simulink model "Basic_DMT"  (R2014b)
settings: Solver=FixedStepDiscrete  SolverMode=SingleTasking  StartTime=0.0  StopTime=25e-6-14e-9*24  RelTol=1e-3
PreLoadFcn:
  | userName = getenv('UserName');
  | 
  | if strcmp(userName,'Tim')
  | cd C:\Users\Tim\Documents\GitHub\MA_1\Basic_DMT
  | else
  | cd C:\Users\Tim-UML\Documents\GitHub\MA_1\Basic_DMT
  | end
InitFcn:
  | userName = getenv('UserName');
  | 
  | if strcmp(userName,'Tim')
  | cd C:\Users\Tim\Documents\GitHub\MA_1\Basic_DMT
  | else
  | cd C:\Users\Tim-UML\Documents\GitHub\MA_1\Basic_DMT
  | end
values from neighbouring files (symbols this model uses):
  a0 = 0.21194908595403703    (= 0.211949085954)    [initScript.m]
  a1 = 0.576101828091926    (= 0.576101828092)    [initScript.m]
  a2 = a0    (= 0.211949085954)    [initScript.m]
  beta = 1    [initScript.m]
  bitPerSymb = 4    [initScript.m]
  chanDownFact = Tchan/SystemPeriod    [initScript.m]
  fftLen = 16    [initScript.m]
  fftLenActive = fftLenDMT    (= 32)    [initScript.m]
  fftLenDMT = 2*fftLen    (= 32)    [initScript.m]
  GI_Active = GI_LenDMT    (= 0)    [initScript.m]
  GI_Len = 0    [initScript.m]
  GI_LenDMT = 0    [initScript.m]
  M = log2(fftLen)    [initScript.m]
  sysgenSystemPeriod = 4e-9    (= 4e-09)    [initScript.m]
  SystemPeriod = 4e-9    (= 4e-09)    [initScript.m]
  upsampleFactor = 1    [initScript.m]
  usedSubCar = 14    [initScript.m]
undefined symbols (not defined in the file or in its folder): bitCount, get, modu_mode, Tb, Ts
libraries: xbsIndex_r4 x822, commdigbbndam3 x59, simulink x42, dspsigops x7, commrandsrc2 x6, dspbuff3 x4, dspxfrm3 x3, dspswit3 x2, commseqgen2 x1, dsparch4 x1, commutil2 x1, dspsnks4 x1
(part 3 of 10)

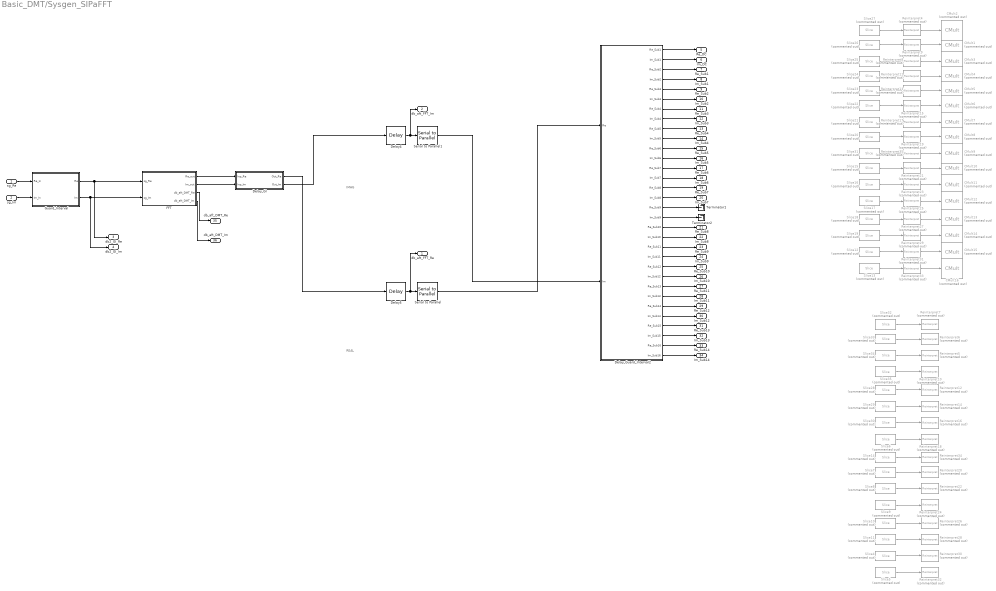
== system Basic_DMT/Sysgen_SIPaFFT ==
  note: IMAG
  note: REAL
  sg_Re : Inport
  sg_Im : Inport  Port=2
  CMult1 : xbsIndex_r4/CMult  Commented=on  const=1/e10  gui_display_data_type=Fixed-point  const_n_bits=bitCount+(log2(fftLen)+1)*2  const_bin_pt=fracLen  float_type=Single  exp_bits=8  fraction_bits=24  en=off  latency=0  precision=User Defined  arith_type="Signed  (2's comp)"  n_bits=bitCount+(log2(fftLen)+1)*2  bin_pt=fracLen  quantization="Round  (unbiased: +/- Inf)"  overflow=Saturate  use_behavioral_HDL=off  mem_type=Distributed RAM  pipeline=off  dbl_ovrd=off  block_type=cmult
  CMult{2,6..16} (12 alike) : xbsIndex_r4/CMult  Commented=on  const=1/e9  gui_display_data_type=Fixed-point  const_n_bits=bitCount+(log2(fftLen)+1)*2  const_bin_pt=fracLen  float_type=Single  exp_bits=8  fraction_bits=24  en=off  latency=0  precision=User Defined  arith_type="Signed  (2's comp)"  n_bits=bitCount+(log2(fftLen)+1)*2  bin_pt=fracLen  quantization="Round  (unbiased: +/- Inf)"  overflow=Saturate  use_behavioral_HDL=off  mem_type=Distributed RAM  pipeline=off  dbl_ovrd=off  block_type=cmult
  CMult3 : xbsIndex_r4/CMult  Commented=on  const=1/e11  gui_display_data_type=Fixed-point  const_n_bits=bitCount+(log2(fftLen)+1)*2  const_bin_pt=fracLen  float_type=Single  exp_bits=8  fraction_bits=24  en=off  latency=0  precision=User Defined  arith_type="Signed  (2's comp)"  n_bits=bitCount+(log2(fftLen)+1)*2  bin_pt=fracLen  quantization="Round  (unbiased: +/- Inf)"  overflow=Saturate  use_behavioral_HDL=off  mem_type=Distributed RAM  pipeline=off  dbl_ovrd=off  block_type=cmult
  CMult4 : xbsIndex_r4/CMult  Commented=on  const=1/e12  gui_display_data_type=Fixed-point  const_n_bits=bitCount+(log2(fftLen)+1)*2  const_bin_pt=fracLen  float_type=Single  exp_bits=8  fraction_bits=24  en=off  latency=0  precision=User Defined  arith_type="Signed  (2's comp)"  n_bits=bitCount+(log2(fftLen)+1)*2  bin_pt=fracLen  quantization="Round  (unbiased: +/- Inf)"  overflow=Saturate  use_behavioral_HDL=off  mem_type=Distributed RAM  pipeline=off  dbl_ovrd=off  block_type=cmult
  CMult5 : xbsIndex_r4/CMult  Commented=on  const=1/e13  gui_display_data_type=Fixed-point  const_n_bits=bitCount+(log2(fftLen)+1)*2  const_bin_pt=fracLen  float_type=Single  exp_bits=8  fraction_bits=24  en=off  latency=0  precision=User Defined  arith_type="Signed  (2's comp)"  n_bits=bitCount+(log2(fftLen)+1)*2  bin_pt=fracLen  quantization="Round  (unbiased: +/- Inf)"  overflow=Saturate  use_behavioral_HDL=off  mem_type=Distributed RAM  pipeline=off  dbl_ovrd=off  block_type=cmult
  Delay4 : xbsIndex_r4/Delay  rst=off  infoeditControl=Selection of Reset will increase slice count due to use of real FFs and instead of SRLs  en=off  latency=4  reg_retiming=off  dbl_ovrd=off  block_type=delay
  Delay5 : xbsIndex_r4/Delay  rst=off  infoeditControl=Selection of Reset will increase slice count due to use of real FFs and instead of SRLs  en=off  latency=4  reg_retiming=off  dbl_ovrd=off  block_type=delay
  Delay_GI : Subsystem  Variant=on
  Delay_Guard_Interval2 : Subsystem  Variant=on
  FFT : Subsystem  Variant=on
  Guard_Interval : Subsystem  Variant=on
  Reinterpret{4..35} (32 alike) : xbsIndex_r4/Reinterpret  Commented=on  force_arith_type=on  arith_type="Signed  (2's comp)"  force_bin_pt=on  bin_pt=fracLen  block_type=reinterpret
  Serial to Parallel : xbsIndex_r4/Serial to Parallel  input_order=Most Significant Word First  arith_type=Unsigned  output_bits=(bitCount+(log2(fftLen)+1)*2)*fftLen  bin_pt=0  rst=off  en=off  latency=1  dbl_ovrd=off  block_type=s2p
      settings: infoedit=Groups of samples presented serially at the input become single samples presented at the output.
  Serial to Parallel1 : xbsIndex_r4/Serial to Parallel  input_order=Most Significant Word First  arith_type=Unsigned  output_bits=(bitCount+(log2(fftLen)+1)*2)*fftLen  bin_pt=0  rst=off  en=off  latency=1  dbl_ovrd=off  block_type=s2p
      settings: infoedit=Groups of samples presented serially at the input become single samples presented at the output.
  Slice10 : xbsIndex_r4/Slice  Commented=on  nbits=(bitCount+(log2(fftLen)+1)*2)  boolean_output=off  mode=Lower Bit Location + Width  bit1=0  base1=MSB of Input  bit0=(bitCount+(log2(fftLen)+1)*2)*3  base0=LSB of Input  dbl_ovrd=off  block_type=slice
  Slice11 : xbsIndex_r4/Slice  Commented=on  nbits=(bitCount+(log2(fftLen)+1)*2)  boolean_output=off  mode=Lower Bit Location + Width  bit1=0  base1=MSB of Input  bit0=(bitCount+(log2(fftLen)+1)*2)*2  base0=LSB of Input  dbl_ovrd=off  block_type=slice
  Slice12 : xbsIndex_r4/Slice  Commented=on  nbits=(bitCount+(log2(fftLen)+1)*2)  boolean_output=off  mode=Lower Bit Location + Width  bit1=0  base1=MSB of Input  bit0=(bitCount+(log2(fftLen)+1)*2)*1  base0=LSB of Input  dbl_ovrd=off  block_type=slice
  Slice13 : xbsIndex_r4/Slice  Commented=on  nbits=(bitCount+(log2(fftLen)+1)*2)  boolean_output=off  mode=Lower Bit Location + Width  bit1=0  base1=MSB of Input  bit0=0  base0=LSB of Input  dbl_ovrd=off  block_type=slice
  Slice14 : xbsIndex_r4/Slice  Commented=on  nbits=(bitCount+(log2(fftLen)+1)*2)  boolean_output=off  mode=Lower Bit Location + Width  bit1=0  base1=LSB of Input  bit0=(bitCount+(log2(fftLen)+1)*2)*7  base0=LSB of Input  dbl_ovrd=off  block_type=slice
  Slice15 : xbsIndex_r4/Slice  Commented=on  nbits=(bitCount+(log2(fftLen)+1)*2)  boolean_output=off  mode=Lower Bit Location + Width  bit1=24  base1=LSB of Input  bit0=(bitCount+(log2(fftLen)+1)*2)*6  base0=LSB of Input  dbl_ovrd=off  block_type=slice
  Slice16 : xbsIndex_r4/Slice  Commented=on  nbits=(bitCount+(log2(fftLen)+1)*2)  boolean_output=off  mode=Lower Bit Location + Width  bit1=0  base1=MSB of Input  bit0=(bitCount+(log2(fftLen)+1)*2)*5  base0=LSB of Input  dbl_ovrd=off  block_type=slice
  Slice17 : xbsIndex_r4/Slice  Commented=on  nbits=(bitCount+(log2(fftLen)+1)*2)  boolean_output=off  mode=Lower Bit Location + Width  bit1=0  base1=MSB of Input  bit0=(bitCount+(log2(fftLen)+1)*2)*4  base0=LSB of Input  dbl_ovrd=off  block_type=slice
  Slice18 : xbsIndex_r4/Slice  Commented=on  nbits=(bitCount+(log2(fftLen)+1)*2)  boolean_output=off  mode=Lower Bit Location + Width  bit1=0  base1=MSB of Input  bit0=(bitCount+(log2(fftLen)+1)*2)*3  base0=LSB of Input  dbl_ovrd=off  block_type=slice
  Slice19 : xbsIndex_r4/Slice  Commented=on  nbits=(bitCount+(log2(fftLen)+1)*2)  boolean_output=off  mode=Lower Bit Location + Width  bit1=0  base1=MSB of Input  bit0=(bitCount+(log2(fftLen)+1)*2)*2  base0=LSB of Input  dbl_ovrd=off  block_type=slice
  Slice20 : xbsIndex_r4/Slice  Commented=on  nbits=(bitCount+(log2(fftLen)+1)*2)  boolean_output=off  mode=Lower Bit Location + Width  bit1=0  base1=LSB of Input  bit0=(bitCount+(log2(fftLen)+1)*2)*8  base0=LSB of Input  dbl_ovrd=off  block_type=slice
  Slice21 : xbsIndex_r4/Slice  Commented=on  nbits=(bitCount+(log2(fftLen)+1)*2)  boolean_output=off  mode=Lower Bit Location + Width  bit1=0  base1=LSB of Input  bit0=(bitCount+(log2(fftLen)+1)*2)*9  base0=LSB of Input  dbl_ovrd=off  block_type=slice
  Slice22 : xbsIndex_r4/Slice  Commented=on  nbits=(bitCount+(log2(fftLen)+1)*2)  boolean_output=off  mode=Lower Bit Location + Width  bit1=0  base1=LSB of Input  bit0=(bitCount+(log2(fftLen)+1)*2)*10  base0=LSB of Input  dbl_ovrd=off  block_type=slice
  Slice23 : xbsIndex_r4/Slice  Commented=on  nbits=(bitCount+(log2(fftLen)+1)*2)  boolean_output=off  mode=Lower Bit Location + Width  bit1=0  base1=LSB of Input  bit0=(bitCount+(log2(fftLen)+1)*2)*11  base0=LSB of Input  dbl_ovrd=off  block_type=slice
  Slice24 : xbsIndex_r4/Slice  Commented=on  nbits=(bitCount+(log2(fftLen)+1)*2)  boolean_output=off  mode=Lower Bit Location + Width  bit1=0  base1=LSB of Input  bit0=(bitCount+(log2(fftLen)+1)*2)*12  base0=LSB of Input  dbl_ovrd=off  block_type=slice
  Slice25 : xbsIndex_r4/Slice  Commented=on  nbits=(bitCount+(log2(fftLen)+1)*2)  boolean_output=off  mode=Lower Bit Location + Width  bit1=0  base1=LSB of Input  bit0=(bitCount+(log2(fftLen)+1)*2)*13  base0=LSB of Input  dbl_ovrd=off  block_type=slice
  Slice26 : xbsIndex_r4/Slice  Commented=on  nbits=(bitCount+(log2(fftLen)+1)*2)  boolean_output=off  mode=Lower Bit Location + Width  bit1=0  base1=LSB of Input  bit0=(bitCount+(log2(fftLen)+1)*2)*14  base0=LSB of Input  dbl_ovrd=off  block_type=slice
  Slice27 : xbsIndex_r4/Slice  Commented=on  nbits=(bitCount+(log2(fftLen)+1)*2)  boolean_output=off  mode=Lower Bit Location + Width  bit1=0  base1=LSB of Input  bit0=(bitCount+(log2(fftLen)+1)*2)*15  base0=LSB of Input  dbl_ovrd=off  block_type=slice
  Slice28 : xbsIndex_r4/Slice  Commented=on  nbits=(bitCount+(log2(fftLen)+1)*2)  boolean_output=off  mode=Lower Bit Location + Width  bit1=0  base1=MSB of Input  bit0=(bitCount+(log2(fftLen)+1)*2)*11  base0=LSB of Input  dbl_ovrd=off  block_type=slice
  Slice29 : xbsIndex_r4/Slice  Commented=on  nbits=(bitCount+(log2(fftLen)+1)*2)  boolean_output=off  mode=Lower Bit Location + Width  bit1=0  base1=MSB of Input  bit0=(bitCount+(log2(fftLen)+1)*2)*10  base0=LSB of Input  dbl_ovrd=off  block_type=slice
  Slice30 : xbsIndex_r4/Slice  Commented=on  nbits=(bitCount+(log2(fftLen)+1)*2)  boolean_output=off  mode=Lower Bit Location + Width  bit1=0  base1=MSB of Input  bit0=(bitCount+(log2(fftLen)+1)*2)*9  base0=LSB of Input  dbl_ovrd=off  block_type=slice
  Slice31 : xbsIndex_r4/Slice  Commented=on  nbits=(bitCount+(log2(fftLen)+1)*2)  boolean_output=off  mode=Lower Bit Location + Width  bit1=0  base1=LSB of Input  bit0=(bitCount+(log2(fftLen)+1)*2)*7  base0=LSB of Input  dbl_ovrd=off  block_type=slice
  Slice32 : xbsIndex_r4/Slice  Commented=on  nbits=(bitCount+(log2(fftLen)+1)*2)  boolean_output=off  mode=Lower Bit Location + Width  bit1=0  base1=LSB of Input  bit0=(bitCount+(log2(fftLen)+1)*2)*15  base0=LSB of Input  dbl_ovrd=off  block_type=slice
  Slice33 : xbsIndex_r4/Slice  Commented=on  nbits=(bitCount+(log2(fftLen)+1)*2)  boolean_output=off  mode=Lower Bit Location + Width  bit1=24  base1=LSB of Input  bit0=(bitCount+(log2(fftLen)+1)*2)*14  base0=LSB of Input  dbl_ovrd=off  block_type=slice
  Slice34 : xbsIndex_r4/Slice  Commented=on  nbits=(bitCount+(log2(fftLen)+1)*2)  boolean_output=off  mode=Lower Bit Location + Width  bit1=0  base1=MSB of Input  bit0=(bitCount+(log2(fftLen)+1)*2)*13  base0=LSB of Input  dbl_ovrd=off  block_type=slice
  Slice35 : xbsIndex_r4/Slice  Commented=on  nbits=(bitCount+(log2(fftLen)+1)*2)  boolean_output=off  mode=Lower Bit Location + Width  bit1=0  base1=MSB of Input  bit0=(bitCount+(log2(fftLen)+1)*2)*12  base0=LSB of Input  dbl_ovrd=off  block_type=slice
  Slice4 : xbsIndex_r4/Slice  Commented=on  nbits=(bitCount+(log2(fftLen)+1)*2)  boolean_output=off  mode=Lower Bit Location + Width  bit1=0  base1=MSB of Input  bit0=(bitCount+(log2(fftLen)+1)*2)  base0=LSB of Input  dbl_ovrd=off  block_type=slice
  Slice5 : xbsIndex_r4/Slice  Commented=on  nbits=(bitCount+(log2(fftLen)+1)*2)  boolean_output=off  mode=Lower Bit Location + Width  bit1=0  base1=MSB of Input  bit0=0  base0=LSB of Input  dbl_ovrd=off  block_type=slice
  Slice6 : xbsIndex_r4/Slice  Commented=on  nbits=(bitCount+(log2(fftLen)+1)*2)  boolean_output=off  mode=Lower Bit Location + Width  bit1=0  base1=LSB of Input  bit0=(bitCount+(log2(fftLen)+1)*2)*8  base0=LSB of Input  dbl_ovrd=off  block_type=slice
  Slice7 : xbsIndex_r4/Slice  Commented=on  nbits=(bitCount+(log2(fftLen)+1)*2)  boolean_output=off  mode=Lower Bit Location + Width  bit1=24  base1=LSB of Input  bit0=(bitCount+(log2(fftLen)+1)*2)*6  base0=LSB of Input  dbl_ovrd=off  block_type=slice
  Slice8 : xbsIndex_r4/Slice  Commented=on  nbits=(bitCount+(log2(fftLen)+1)*2)  boolean_output=off  mode=Lower Bit Location + Width  bit1=0  base1=MSB of Input  bit0=(bitCount+(log2(fftLen)+1)*2)*5  base0=LSB of Input  dbl_ovrd=off  block_type=slice
  Slice9 : xbsIndex_r4/Slice  Commented=on  nbits=(bitCount+(log2(fftLen)+1)*2)  boolean_output=off  mode=Lower Bit Location + Width  bit1=0  base1=MSB of Input  bit0=(bitCount+(log2(fftLen)+1)*2)*4  base0=LSB of Input  dbl_ovrd=off  block_type=slice
  Terminator1 : Terminator
  Terminator2 : Terminator
  db_aft_FFT_Re : Outport
  db_aft_FFT_Im : Outport  Port=2
  db2_GI_Re : Outport  Port=3
  db2_GI_Im : Outport  Port=4
  Re_DC : Outport  Port=5
  Im_DC : Outport  Port=6
  Re_Sub1 : Outport  Port=7
  Im_Sub1 : Outport  Port=8
  Re_Sub2 : Outport  Port=9
  Im_Sub2 : Outport  Port=10
  Re_Sub3 : Outport  Port=11
  Im_Sub3 : Outport  Port=12
  Re_Sub4 : Outport  Port=13
  Im_Sub4 : Outport  Port=14
  Re_Sub5 : Outport  Port=15
  Im_Sub5 : Outport  Port=16
  Re_Sub6 : Outport  Port=17
  Im_Sub6 : Outport  Port=18
  Re_Sub7 : Outport  Port=19
  Im_Sub7 : Outport  Port=20
  Re_Sub8 : Outport  Port=21
  Im_Sub8 : Outport  Port=22
  Re_Sub9 : Outport  Port=23
  Im_Sub9 : Outport  Port=24
  Re_Sub10 : Outport  Port=25
  Im_Sub10 : Outport  Port=26
  Re_Sub11 : Outport  Port=27
  Im_Sub11 : Outport  Port=28
  Re_Sub12 : Outport  Port=29
  Im_Sub12 : Outport  Port=30
  Re_Sub13 : Outport  Port=31
  Im_Sub13 : Outport  Port=32
  Re_Sub14 : Outport  Port=33
  Im_Sub14 : Outport  Port=34
  db_aft_DMT_Re : Outport  Port=35
  db_aft_DMT_Im : Outport  Port=36
  wires:
  Delay_Guard_Interval2/1(Re_Sub1) -> Re_DC/1
  Delay_Guard_Interval2/3(Re_Sub2) -> Re_Sub1/1
  Delay4/1 -> db_aft_FFT_Im/1, Serial to Parallel1/1
  Delay5/1 -> db_aft_FFT_Re/1, Serial to Parallel/1
  Delay_Guard_Interval2/5(Re_Sub3) -> Re_Sub2/1
  Guard_Interval/1(Re) -> FFT/1(sg_Re), db2_GI_Re/1
  Guard_Interval/2(Im) -> FFT/2(sg_Im), db2_GI_Im/1
  sg_Im/1 -> Guard_Interval/2(Im_In)
  sg_Re/1 -> Guard_Interval/1(Re_In)
  Delay_Guard_Interval2/7(Re_Sub4) -> Re_Sub3/1
  Delay_Guard_Interval2/9(Re_Sub5) -> Re_Sub4/1
  Delay_Guard_Interval2/11(Re_Sub6) -> Re_Sub5/1
  Delay_Guard_Interval2/15(Re_Sub8) -> Re_Sub7/1
  Delay_Guard_Interval2/13(Re_Sub7) -> Re_Sub6/1
  Delay_Guard_Interval2/23(Re_Sub12) -> Re_Sub10/1
  Delay_Guard_Interval2/19(Re_Sub10) -> Re_Sub8/1
  Delay_Guard_Interval2/21(Re_Sub11) -> Re_Sub9/1
  Delay_Guard_Interval2/25(Re_Sub13) -> Re_Sub11/1
  Delay_Guard_Interval2/27(Re_Sub14) -> Re_Sub12/1
  Delay_Guard_Interval2/29(Re_Sub15) -> Re_Sub13/1
  Delay_Guard_Interval2/31(Re_Sub16) -> Re_Sub14/1
  Serial to Parallel/1 -> Delay_Guard_Interval2/1(Re)
  Delay_Guard_Interval2/17(Re_Sub9) -> Terminator1/1
  Delay_GI/2(Out_Im) -> Delay4/1
  Delay_GI/1(Out_Re) -> Delay5/1
  FFT/3(db_aft_DMT_Re) -> db_aft_DMT_Re/1
  FFT/4(db_aft_DMT_Im) -> db_aft_DMT_Im/1
  FFT/1(Re_out) -> Delay_GI/1(Inp_Re)
  FFT/2(Im_out) -> Delay_GI/2(Inp_Im)
  Delay_Guard_Interval2/2(Im_Sub1) -> Im_DC/1
  Delay_Guard_Interval2/4(Im_Sub2) -> Im_Sub1/1
  Delay_Guard_Interval2/6(Im_Sub3) -> Im_Sub2/1
  Delay_Guard_Interval2/8(Im_Sub4) -> Im_Sub3/1
  Delay_Guard_Interval2/10(Im_Sub5) -> Im_Sub4/1
  Delay_Guard_Interval2/12(Im_Sub6) -> Im_Sub5/1
  Delay_Guard_Interval2/14(Im_Sub7) -> Im_Sub6/1
  Delay_Guard_Interval2/16(Im_Sub8) -> Im_Sub7/1
  Delay_Guard_Interval2/18(Im_Sub9) -> Terminator2/1
  Delay_Guard_Interval2/20(Im_Sub10) -> Im_Sub8/1
  Delay_Guard_Interval2/22(Im_Sub11) -> Im_Sub9/1
  Delay_Guard_Interval2/24(Im_Sub12) -> Im_Sub10/1
  Delay_Guard_Interval2/26(Im_Sub13) -> Im_Sub11/1
  Delay_Guard_Interval2/28(Im_Sub14) -> Im_Sub12/1
  Delay_Guard_Interval2/30(Im_Sub15) -> Im_Sub13/1
  Delay_Guard_Interval2/32(Im_Sub16) -> Im_Sub14/1
  Reinterpret4/1 -> CMult2/1
  Reinterpret9/1 -> CMult1/1
  Reinterpret8/1 -> CMult3/1
  Slice26/1 -> Reinterpret9/1
  Slice27/1 -> Reinterpret4/1
  Reinterpret11/1 -> CMult4/1
  Reinterpret13/1 -> CMult5/1
  Reinterpret15/1 -> CMult6/1
  Reinterpret17/1 -> CMult7/1
  Reinterpret19/1 -> CMult8/1
  Reinterpret21/1 -> CMult10/1
  Reinterpret23/1 -> CMult11/1
  Reinterpret25/1 -> CMult12/1
  Reinterpret27/1 -> CMult13/1
  Reinterpret29/1 -> CMult14/1
  Reinterpret31/1 -> CMult15/1
  Reinterpret33/1 -> CMult16/1
  Slice25/1 -> Reinterpret8/1
  Slice24/1 -> Reinterpret11/1
  Slice23/1 -> Reinterpret13/1
  Slice22/1 -> Reinterpret15/1
  Slice20/1 -> Reinterpret19/1
  Slice21/1 -> Reinterpret17/1
  Slice15/1 -> Reinterpret21/1
  Slice16/1 -> Reinterpret23/1
  Slice17/1 -> Reinterpret25/1
  Slice18/1 -> Reinterpret27/1
  Slice19/1 -> Reinterpret29/1
  Slice12/1 -> Reinterpret31/1
  Slice13/1 -> Reinterpret33/1
  Slice31/1 -> Reinterpret35/1
  Reinterpret35/1 -> CMult9/1
  Serial to Parallel1/1 -> Delay_Guard_Interval2/2(Im)
  Slice32/1 -> Reinterpret7/1
  Slice33/1 -> Reinterpret6/1
  Slice34/1 -> Reinterpret5/1
  Slice35/1 -> Reinterpret10/1
  Slice28/1 -> Reinterpret12/1
  Slice29/1 -> Reinterpret14/1
  Slice30/1 -> Reinterpret16/1
  Slice7/1 -> Reinterpret20/1
  Slice8/1 -> Reinterpret22/1
  Slice9/1 -> Reinterpret24/1
  Slice10/1 -> Reinterpret26/1
  Slice11/1 -> Reinterpret28/1
  Slice4/1 -> Reinterpret30/1
  Slice5/1 -> Reinterpret32/1
  Slice6/1 -> Reinterpret18/1
  Slice14/1 -> Reinterpret34/1

== system Basic_DMT/Testsystem Channelfilter ==
  Add2 : Sum  Commented=on  Inputs=+-  OutDataTypeStr=Inherit: Same as first input
  AddSub : xbsIndex_r4/AddSub  Commented=on  mode=Addition  use_carryin=off  use_carryout=off  en=off  latency=0  precision=User Defined  arith_type="Signed  (2's comp)"  n_bits=bitCount+(log2(fftLen)+1)  bin_pt=fracLen  quantization="Round  (unbiased: +/- Inf)"  overflow=Saturate  use_behavioral_HDL=off  hw_selection=Fabric  pipelined=off  dbl_ovrd=off  block_type=addsub
  AddSub1 : xbsIndex_r4/AddSub  Commented=on  mode=Addition  use_carryin=off  use_carryout=off  en=off  latency=0  precision=User Defined  arith_type="Signed  (2's comp)"  n_bits=bitCount+(log2(fftLen)+1)  bin_pt=fracLen  quantization="Round  (unbiased: +/- Inf)"  overflow=Saturate  use_behavioral_HDL=off  hw_selection=Fabric  pipelined=off  dbl_ovrd=off  block_type=addsub
  Bernoulli Binary Generator1 : commrandsrc2/Bernoulli Binary Generator  Commented=on  P=0.5  seed=1604198  Ts=Tb  frameBased=off  sampPerFrame=1  orient=off  outDataType=double
      settings: AttributesFormatString=|
      | Sample Time= %<Ts>
      | Prob zero=%<P>
  CMult{,1,4..5} (4 alike) : xbsIndex_r4/CMult  Commented=on  const=.5  gui_display_data_type=Fixed-point  const_n_bits=bitCount+(log2(fftLen)+1)  const_bin_pt=fracLen  float_type=Single  exp_bits=8  fraction_bits=24  en=off  latency=0  precision=User Defined  arith_type="Signed  (2's comp)"  n_bits=bitCount+(log2(fftLen)+1)  bin_pt=fracLen  quantization="Round  (unbiased: +/- Inf)"  overflow=Saturate  use_behavioral_HDL=off  mem_type=Distributed RAM  pipeline=off  dbl_ovrd=off  block_type=cmult
  Data Type Conversion : DataTypeConversion  Commented=on  OutDataTypeStr=fixdt(1,21,13)  RndMeth=Convergent
  Delay2 : xbsIndex_r4/Delay  Commented=on  rst=off  infoeditControl=Selection of Reset will increase slice count due to use of real FFs and instead of SRLs  en=off  latency=1  reg_retiming=off  dbl_ovrd=off  block_type=delay
  Delay3 : xbsIndex_r4/Delay  Commented=on  rst=off  infoeditControl=Selection of Reset will increase slice count due to use of real FFs and instead of SRLs  en=off  latency=1  reg_retiming=off  dbl_ovrd=off  block_type=delay
  Delay4 : xbsIndex_r4/Delay  Commented=on  rst=off  infoeditControl=Selection of Reset will increase slice count due to use of real FFs and instead of SRLs  en=off  latency=15  reg_retiming=off  dbl_ovrd=off  block_type=delay
  Delay5 : Delay  Commented=on  DelayLength=15  InitialCondition=0
  Discrete FIR Filter7 : DiscreteFir  Commented=on  RndMeth=Convergent  SaturateOnIntegerOverflow=on  OutDataTypeStr=Inherit: Same as input
  Discrete FIR Filter8 : DiscreteFir  Commented=on  RndMeth=Convergent  SaturateOnIntegerOverflow=on  OutDataTypeStr=Inherit: Same as input
  Gateway In2 : xbsIndex_r4/Gateway In  Commented=on  gui_display_data_type=Fixed-point  arith_type="Signed  (2's comp)"  n_bits=21  bin_pt=14  preci_type=Single  exp_width=8  frac_width=24  rows=1  columns=1  quantization="Round  (unbiased: +/- Inf)"  overflow=Saturate  period=Ts  UseAsADC=off  ADCChannel='1'  interface=None  automatic_assignment=on  address_offset=hex2dec('00')  intf_description=''  timing_constraint=None  locs_specified=off  LOCs={}  io_standard={}  inherit_from_input=off  hdl_port=on  dbl_ovrd=off  block_type=gatewayin
  Gateway Out1 : xbsIndex_r4/Gateway Out  Commented=on  inherit_from_input=off  hdl_port=on  rows=1  columns=1  UseAsDAC=off  DACChannel='1'  interface=None  automatic_assignment=on  address_offset=hex2dec('00')  intf_description=''  timing_constraint=None  locs_specified=off  LOCs={}  io_standard={}  block_type=gatewayout
  Scope5 : Scope  Commented=on  NumInputPorts=3
      settings: TimeRange=2e-05  YMin=-10~-8~-5  YMax=8~8~5  SaveName=ScopeData50
  wires:
  Delay4/1 -> Gateway Out1/1
  Delay2/1 -> CMult1/1
  Gateway In2/1 -> CMult/1, Delay2/1
  AddSub/1 -> CMult4/1, Delay3/1
  CMult1/1 -> AddSub/1
  CMult4/1 -> AddSub1/2
  AddSub1/1 -> Delay4/1
  CMult/1 -> AddSub/2
  Delay3/1 -> CMult5/1
  CMult5/1 -> AddSub1/1
  Discrete FIR Filter7/1 -> Discrete FIR Filter8/1
  Discrete FIR Filter8/1 -> Delay5/1
  Bernoulli Binary Generator1/1 -> Gateway In2/1, Data Type Conversion/1
  Gateway Out1/1 -> Add2/2, Scope5/2
  Add2/1 -> Scope5/3
  Delay5/1 -> Add2/1, Scope5/1
  Data Type Conversion/1 -> Discrete FIR Filter7/1

== system Basic_DMT/Testsystem to examine Demux ==
  " System Generator" : xbsIndex_r4/ System Generator  Tag=genX  xilinxfamily=zynq  part=xc7z020  speed=-1  package=clg400  synthesis_tool=Vivado  clock_wrapper=Clock Enables  directory=./netlist  proj_type=Vivado  Synth_file=Vivado Synthesis Defaults  Impl_file=Vivado Implementation Defaults  testbench=on  simulink_period=Ts  sysclk_period=10  dcm_input_clock_period=10  incr_netlist=off  trim_vbits=Everywhere in SubSystem  dbl_ovrd=According to Block Masks  core_generation=According to Block Masks  run_coregen=off  deprecated_control=off  eval_field=0  block_type=sysgen
  Bernoulli Binary Generator1 : commrandsrc2/Bernoulli Binary Generator  P=0.5  seed=1604198  Ts=Tb  frameBased=off  sampPerFrame=1  orient=off  outDataType=boolean
      settings: AttributesFormatString=|
      | Sample Time= %<Ts>
      | Prob zero=%<P>
  Buffer : Buffer  N=8  TreatMby1Signals=One channel
  Clock Probe1 : xbsIndex_r4/Clock Probe  block_type=clkprobe
      settings: infoedit="Clock probe.  Produces an output of type double that mirrors the hardware system clock.<br><br>Hardware notes:  This block is ignored when hardware is generated."
  Counter Limited2 : simulink/Sources/Counter Limited  uplimit=1  tsamp=Tb
  Demux : Demux  Outputs=2
  Manual Switch1 : ManualSwitch  CurrentSetting=0
  Scope3 : Scope  NumInputPorts=5
      settings: YMin=-5~-5~-5~-5~-5  YMax=5~5~5~5~5  SaveName=ScopeData5
  Unbuffer1 : Unbuffer  SampleBasedProcessing=Same as frame based
  Unbuffer2 : Unbuffer  SampleBasedProcessing=Same as frame based
  Unbuffer3 : Unbuffer  SampleBasedProcessing=Same as frame based
  wires:
  Bernoulli Binary Generator1/1 -> Manual Switch1/2
  Counter Limited2/1 -> Manual Switch1/1
  Clock Probe1/1 -> Scope3/5
  Unbuffer3/1 -> Scope3/1
  Manual Switch1/1 -> Scope3/4, Buffer/1
  Unbuffer2/1 -> Scope3/3
  Demux/1 -> Unbuffer3/1
  Unbuffer1/1 -> Scope3/2
  Demux/2 -> Unbuffer1/1
  Buffer/1 -> Unbuffer2/1, Demux/1

== system Basic_DMT/Total Bits // Subchannel Information ==
  Display : Display
  Display1 : Display
  Sub-Channel-Information : MATLAB Function  TreatAsAtomicUnit=on
  "Total-Bits " : MATLAB Function  TreatAsAtomicUnit=on
  wires:
  "Total-Bits "/1(y) -> Display1/1
  Sub-Channel-Information/1(y) -> "Total-Bits "/1(x), Display/1

== system Basic_DMT/Transmitter ==

== system Basic_DMT/Versuche DEMUX verm. löschen ==
  Buffer : Buffer  Commented=on  N=2  TreatMby1Signals=One channel
  Clock Probe : xbsIndex_r4/Clock Probe  Commented=on  block_type=clkprobe
      settings: infoedit="Clock probe.  Produces an output of type double that mirrors the hardware system clock.<br><br>Hardware notes:  This block is ignored when hardware is generated."
  Counter Limited : simulink/Sources/Counter Limited  Commented=on  uplimit=7  tsamp=Ts
  Counter1 : xbsIndex_r4/Counter  Commented=on  cnt_type=Count Limited  cnt_to=7  operation=Up  start_count=0  cnt_by_val=1  arith_type=Unsigned  n_bits=8  bin_pt=0  load_pin=off  rst=off  en=off  explicit_period=on  period=Ts  use_behavioral_HDL=off  implementation=Fabric  dbl_ovrd=off  block_type=counter
  Counter2 : xbsIndex_r4/Counter  Commented=on  cnt_type=Count Limited  cnt_to=7  operation=Up  start_count=0  cnt_by_val=1  arith_type=Unsigned  n_bits=8  bin_pt=0  load_pin=off  rst=off  en=off  explicit_period=on  period=Ts  use_behavioral_HDL=off  implementation=Fabric  dbl_ovrd=off  block_type=counter
  Demux : Demux  Commented=on  Outputs=2
  Down Sample : xbsIndex_r4/Down Sample  Commented=on  sample_ratio=2  sample_phase=First Value of Frame  en=off  rst=off  latency=0  dbl_ovrd=off  block_type=dsamp
  Gateway In : xbsIndex_r4/Gateway In  Commented=on  gui_display_data_type=Boolean  arith_type=Boolean  n_bits=16  bin_pt=14  preci_type=Single  exp_width=8  frac_width=24  rows=1  columns=1  quantization="Round  (unbiased: +/- Inf)"  overflow=Saturate  period=Ts  UseAsADC=off  ADCChannel='1'  interface=None  automatic_assignment=on  address_offset=hex2dec('00')  intf_description=''  timing_constraint=None  locs_specified=off  LOCs={}  io_standard={}  inherit_from_input=off  hdl_port=on  dbl_ovrd=off  block_type=gatewayin
  Gateway Out{,1..3} (4 alike) : xbsIndex_r4/Gateway Out  Commented=on  inherit_from_input=on  hdl_port=off  rows=1  columns=1  UseAsDAC=off  DACChannel='1'  interface=None  automatic_assignment=on  address_offset=hex2dec('00')  intf_description=''  timing_constraint=None  locs_specified=off  LOCs={}  io_standard={}  block_type=gatewayout
  MCode : xbsIndex_r4/MCode  Commented=on  mfname=xlmax  explicit_period=on  period=Ts*2  inputsTable={'boundInpExpr'=>['',''],'inputs'=>['x1','x2']}  outputsTable={'outputs'=>['y1','y2'],'suppressOut'=>['off','off']}  enable_stdout=off  enable_debug=off  suppress_output=on  defparams={}  hide_port_list={}  dbl_ovrd=off  block_type=mcode
  Register : xbsIndex_r4/Register  Commented=on  init=0  rst=off  en=off  dbl_ovrd=off  block_type=register
  Register1 : xbsIndex_r4/Register  Commented=on  init=0  rst=off  en=off  dbl_ovrd=off  block_type=register
  Register2 : xbsIndex_r4/Register  Commented=on  init=0  rst=off  en=on  dbl_ovrd=off  block_type=register
  Register3 : xbsIndex_r4/Register  Commented=on  init=0  rst=off  en=on  dbl_ovrd=off  block_type=register
  Scope3 : Scope  Commented=on  NumInputPorts=5
      settings: YMin=-5~-5~-5~-5~-5  YMax=5~5~5~5~5  SaveName=ScopeData7
  Subtract : Sum  Commented=on  Inputs=+-
  Out1 : Outport
  Out2 : Outport  Port=2
  wires:
  Register1/1 -> MCode/1
  Subtract/1 -> Scope3/3
  ? -> Gateway Out1/1
  MCode/1 -> Gateway Out/1
  Buffer/1 -> Demux/1
  Counter2/1 -> Register2/1
  Gateway Out/1 -> Subtract/1, Scope3/1
  Demux/1 -> Scope3/2, Subtract/2
  Counter1/1 -> Register/1
  Register/1 -> Register1/1
  Counter Limited/1 -> Buffer/1
  Down Sample/1 -> Register2/2, Register3/2
  Clock Probe/1 -> Gateway In/1
  Gateway In/1 -> Down Sample/1
  Register2/1 -> Gateway Out3/1, Register3/1
  Register3/1 -> Gateway Out2/1
  Gateway Out3/1 -> Scope3/5
  Gateway Out2/1 -> Scope3/4
  Gateway Out1/1 -> Out1/1
  Demux/2 -> Out2/1

== system Basic_DMT/16-QAM Sysgen/16-QAM ==
  In1 : Inport
  BitBasher : xbsIndex_r4/BitBasher  bitexpr=|  display_expr=on  sr_1=b  arith_type1=Unsigned  bin_pt1=0  sr_2=c  arith_type2=Unsigned  bin_pt2=0  sr_3=3  arith_type3=Unsigned  bin_pt3=0  sr_4=4  arith_type4=Unsigned  bin_pt4=0  dbl_ovrd=off  block_type=bitbasher
      | b={a[3:2]}
      | c={a[1:0]}
  Constant1 : xbsIndex_r4/Constant  const=-3  gui_display_data_type=Floating-point  arith_type=Floating-point  n_bits=16  bin_pt=14  preci_type=Single  exp_width=8  frac_width=24  explicit_period=off  period=Ts  equ=P=C  opselect=C  inp2=PCIN>>17  opr=+  inp1=P  carry=CIN  dbl_ovrd=off  block_type=constant
  Constant2 : xbsIndex_r4/Constant  const=-1  gui_display_data_type=Floating-point  arith_type=Floating-point  n_bits=16  bin_pt=14  preci_type=Single  exp_width=8  frac_width=24  explicit_period=off  period=Ts  equ=P=C  opselect=C  inp2=PCIN>>17  opr=+  inp1=P  carry=CIN  dbl_ovrd=off  block_type=constant
  Constant3 : xbsIndex_r4/Constant  const=3  gui_display_data_type=Floating-point  arith_type=Floating-point  n_bits=16  bin_pt=14  preci_type=Single  exp_width=8  frac_width=24  explicit_period=off  period=Ts  equ=P=C  opselect=C  inp2=PCIN>>17  opr=+  inp1=P  carry=CIN  dbl_ovrd=off  block_type=constant
  Constant4 : xbsIndex_r4/Constant  const=1  gui_display_data_type=Floating-point  arith_type=Floating-point  n_bits=16  bin_pt=14  preci_type=Single  exp_width=8  frac_width=24  explicit_period=off  period=Ts  equ=P=C  opselect=C  inp2=PCIN>>17  opr=+  inp1=P  carry=CIN  dbl_ovrd=off  block_type=constant
  Constant5 : xbsIndex_r4/Constant  const=3  gui_display_data_type=Floating-point  arith_type=Floating-point  n_bits=16  bin_pt=14  preci_type=Single  exp_width=8  frac_width=24  explicit_period=off  period=Ts  equ=P=C  opselect=C  inp2=PCIN>>17  opr=+  inp1=P  carry=CIN  dbl_ovrd=off  block_type=constant
  Constant6 : xbsIndex_r4/Constant  const=1  gui_display_data_type=Floating-point  arith_type=Floating-point  n_bits=16  bin_pt=14  preci_type=Single  exp_width=8  frac_width=24  explicit_period=off  period=Ts  equ=P=C  opselect=C  inp2=PCIN>>17  opr=+  inp1=P  carry=CIN  dbl_ovrd=off  block_type=constant
  Constant7 : xbsIndex_r4/Constant  const=-3  gui_display_data_type=Floating-point  arith_type=Floating-point  n_bits=16  bin_pt=14  preci_type=Single  exp_width=8  frac_width=24  explicit_period=off  period=Ts  equ=P=C  opselect=C  inp2=PCIN>>17  opr=+  inp1=P  carry=CIN  dbl_ovrd=off  block_type=constant
  Constant8 : xbsIndex_r4/Constant  const=-1  gui_display_data_type=Floating-point  arith_type=Floating-point  n_bits=16  bin_pt=14  preci_type=Single  exp_width=8  frac_width=24  explicit_period=off  period=Ts  equ=P=C  opselect=C  inp2=PCIN>>17  opr=+  inp1=P  carry=CIN  dbl_ovrd=off  block_type=constant
  Mux : xbsIndex_r4/Mux  inputs=4  en=off  latency=1  precision=Full  arith_type=Unsigned  n_bits=16  bin_pt=14  quantization=Truncate  overflow=Wrap  dbl_ovrd=off  block_type=mux
  Mux1 : xbsIndex_r4/Mux  inputs=4  en=off  latency=1  precision=Full  arith_type=Unsigned  n_bits=16  bin_pt=14  quantization=Truncate  overflow=Wrap  dbl_ovrd=off  block_type=mux
  Out2 : Outport
  Out3 : Outport  Port=2
  wires:
  Mux1/1 -> Out3/1
  In1/1 -> BitBasher/1
  Constant1/1 -> Mux/2
  Constant2/1 -> Mux/3
  BitBasher/1 -> Mux/1
  Constant5/1 -> Mux1/2
  Constant6/1 -> Mux1/3
  Constant8/1 -> Mux1/5
  Constant7/1 -> Mux1/4
  BitBasher/2 -> Mux1/1
  Constant4/1 -> Mux/5
  Mux/1 -> Out2/1
  Constant3/1 -> Mux/4

== system Basic_DMT/AWGN/No_AWGN ==
  sig_in : Inport
  db_bool : Inport  Port=2
  db_full : Inport  Port=3
  Terminator : Terminator
  Terminator1 : Terminator
  sig_out : Outport
  wires:
  sig_in/1 -> sig_out/1
  db_full/1 -> Terminator/1
  db_bool/1 -> Terminator1/1

== system Basic_DMT/AWGN/Yes_AWGN ==
  sig_in : Inport
  db_bool : Inport  Port=2
  db_full : Inport  Port=3
  Add1 : Sum  Inputs=+-  OutDataTypeStr=Inherit: Same as first input
  Add2 : Sum  OutDataTypeStr=Inherit: Same as first input
  Add3 : Sum  OutDataTypeStr=Inherit: Same as first input
  Add4 : Sum  Inputs=+-  RndMeth=Convergent  OutDataTypeStr=Inherit: Same as first input
  Add5 : Sum  Inputs=+-  OutDataTypeStr=Inherit: Same as first input
  Complex to Real-Imag2 : ComplexToRealImag
  Constant1 : Constant  Value=0.5  OutDataTypeStr=Inherit: Inherit via back propagation
  Data_Type_Conversion : DataTypeConversion  OutDataTypeStr=double  RndMeth=Convergent
  Delay : Delay  DelayLength=1
  Delay2 : Delay  DelayLength=1
  Delay3 : Delay  DelayLength=1
  Delay4 : Delay  Commented=through  DelayLength=1
  Discrete-Time Integrator : DiscreteIntegrator  InitialConditionSetting=State (most efficient)  SampleTime=-1
  Gain : Gain  Gain=1.58*2  RndMeth=Convergent  OutDataTypeStr=Inherit: Same as input
  Gateway Out1 : xbsIndex_r4/Gateway Out  inherit_from_input=off  hdl_port=off  rows=1  columns=1  UseAsDAC=off  DACChannel='1'  interface=None  automatic_assignment=on  address_offset=hex2dec('00')  intf_description=''  timing_constraint=None  locs_specified=off  LOCs={}  io_standard={}  block_type=gatewayout
  Gateway Out2 : xbsIndex_r4/Gateway Out  inherit_from_input=on  hdl_port=off  rows=1  columns=1  UseAsDAC=off  DACChannel='1'  interface=None  automatic_assignment=on  address_offset=hex2dec('00')  intf_description=''  timing_constraint=None  locs_specified=off  LOCs={}  io_standard={}  block_type=gatewayout
  PN_Sequence_Generator : commseqgen2/PN Sequence Generator  poly=[1 0 0 0 0 1 1]  ini_sta=[0 0 0 0 0 1]  outBitMaskSource=Dialog parameter  shift=[1 1 0 1 0 1]  outVarSiz=off  maxOutSizeMode=Dialog parameter  maxOutSize=[10 1]  Ts=bitPerSymb*usedSubCar*Ts/(fftLenActive+GI_Active)/upsampleFactor  frameBased=off  sampPerFrame=1  reset=off  bitPackedOutputs=off  outDataType=double  numPackedBits=8  bitPackDataSigned=off  bitPackedOutDType=double
  Real-Imag to Complex : RealImagToComplex
  Scope1 : Scope  Commented=on
      settings: YMin=-10  YMax=8  SaveName=ScopeData52
  Scope2 : Scope  NumInputPorts=3
      settings: TimeRange=2e-05  YMin=-10~-8~-5  YMax=8~8~5  SaveName=ScopeData53
  Scope5 : Scope  Commented=on  NumInputPorts=3
      settings: TimeRange=2e-05  YMin=-10~-8~-5  YMax=8~8~5  SaveName=ScopeData54
  sig_out : Outport
  wires:
  sig_in/1 -> Complex to Real-Imag2/1
  Real-Imag to Complex/1 -> Delay4/1
  Data_Type_Conversion/1 -> Delay/1
  Constant1/1 -> Add4/2
  Add3/1 -> Real-Imag to Complex/1
  PN_Sequence_Generator/1 -> Add1/1, Scope5/1, Data_Type_Conversion/1
  Complex to Real-Imag2/2 -> Add2/1
  Add2/1 -> Real-Imag to Complex/2
  Complex to Real-Imag2/1 -> Add3/1
  Add4/1 -> Delay2/1
  Gain/1 -> Delay3/1
  Discrete-Time Integrator/1 -> Scope1/1
  Gateway Out2/1 -> Add1/2, Scope5/2
  Add1/1 -> Scope5/3
  Delay/1 -> Add4/1
  Delay2/1 -> Gain/1
  Delay3/1 -> Add5/1, Scope2/1, Discrete-Time Integrator/1, Add3/2, Add2/2
  Gateway Out1/1 -> Add5/2, Scope2/2
  Add5/1 -> Scope2/3
  db_bool/1 -> Gateway Out2/1
  db_full/1 -> Gateway Out1/1
  Delay4/1 -> sig_out/1

== system Basic_DMT/Channel/No_channel ==
  sig_in : Inport
  db_Re : Inport  Port=2
  Delay : Delay  DelayLength=(fftLen+GI_Len)*upsampleFactor  InitialCondition=0
  Terminator : Terminator
  sig_out : Outport
  wires:
  sig_in/1 -> Delay/1
  Delay/1 -> sig_out/1
  db_Re/1 -> Terminator/1

== system Basic_DMT/Channel/Yes_Channel ==
  sig_in : Inport
  db_Re : Inport  Port=2
  Add3 : Sum  Inputs=+-
  Complex to Real-Imag : ComplexToRealImag
  Delay1 : Delay  DelayLength=(fftLen-1+GI_Len)*upsampleFactor  InitialCondition=0
  Delay_upsample : Subsystem  Variant=on
  Discrete FIR Filter1 : DiscreteFir  Commented=on  RndMeth=Convergent  SaturateOnIntegerOverflow=on  OutDataTypeStr=Inherit: Same as input
  Discrete FIR Filter2 : DiscreteFir  Commented=on  Coefficients=[0.5 +0.5]  RndMeth=Convergent  SaturateOnIntegerOverflow=on  OutDataTypeStr=Inherit: Same as input
  Discrete FIR Filter4 : DiscreteFir  Coefficients=[a0 a1 a2]  RndMeth=Convergent  SaturateOnIntegerOverflow=on  OutDataTypeStr=Inherit: Same as input
  Gateway Out : xbsIndex_r4/Gateway Out  inherit_from_input=off  hdl_port=off  rows=1  columns=1  UseAsDAC=off  DACChannel='1'  interface=None  automatic_assignment=on  address_offset=hex2dec('00')  intf_description=''  timing_constraint=None  locs_specified=off  LOCs={}  io_standard={}  block_type=gatewayout
  Scope12 : Scope  NumInputPorts=3
      settings: YMin=-5~-5~-5  YMax=5~5~5  SaveName=ScopeData48
  Terminator : Terminator
  sig_out : Outport
  wires:
  Discrete FIR Filter4/1 -> Delay1/1
  sig_in/1 -> Discrete FIR Filter4/1
  Delay1/1 -> Delay_upsample/1(In1)
  Delay_upsample/1(Out1) -> Complex to Real-Imag/1, sig_out/1
  Add3/1 -> Scope12/3
  Gateway Out/1 -> Add3/2, Scope12/2
  db_Re/1 -> Gateway Out/1
  Complex to Real-Imag/1 -> Add3/1, Scope12/1
  Complex to Real-Imag/2 -> Terminator/1
  Discrete FIR Filter1/1 -> Discrete FIR Filter2/1

== system Basic_DMT/Combination of Sysgen S//P and 16QAM/16-QAM 1 ==
  In1 : Inport
  BitBasher : xbsIndex_r4/BitBasher  bitexpr=|  display_expr=on  sr_1=b  arith_type1=Unsigned  bin_pt1=0  sr_2=c  arith_type2=Unsigned  bin_pt2=0  sr_3=3  arith_type3=Unsigned  bin_pt3=0  sr_4=4  arith_type4=Unsigned  bin_pt4=0  dbl_ovrd=off  block_type=bitbasher
      | b={a[3:2]}
      | c={a[1:0]}
  Constant1 : xbsIndex_r4/Constant  const=-3  gui_display_data_type=Floating-point  arith_type=Floating-point  n_bits=16  bin_pt=14  preci_type=Single  exp_width=8  frac_width=24  explicit_period=off  period=Ts  equ=P=C  opselect=C  inp2=PCIN>>17  opr=+  inp1=P  carry=CIN  dbl_ovrd=off  block_type=constant
  Constant2 : xbsIndex_r4/Constant  const=-1  gui_display_data_type=Floating-point  arith_type=Floating-point  n_bits=16  bin_pt=14  preci_type=Single  exp_width=8  frac_width=24  explicit_period=off  period=Ts  equ=P=C  opselect=C  inp2=PCIN>>17  opr=+  inp1=P  carry=CIN  dbl_ovrd=off  block_type=constant
  Constant3 : xbsIndex_r4/Constant  const=3  gui_display_data_type=Floating-point  arith_type=Floating-point  n_bits=16  bin_pt=14  preci_type=Single  exp_width=8  frac_width=24  explicit_period=off  period=Ts  equ=P=C  opselect=C  inp2=PCIN>>17  opr=+  inp1=P  carry=CIN  dbl_ovrd=off  block_type=constant
  Constant4 : xbsIndex_r4/Constant  const=1  gui_display_data_type=Floating-point  arith_type=Floating-point  n_bits=16  bin_pt=14  preci_type=Single  exp_width=8  frac_width=24  explicit_period=off  period=Ts  equ=P=C  opselect=C  inp2=PCIN>>17  opr=+  inp1=P  carry=CIN  dbl_ovrd=off  block_type=constant
  Constant5 : xbsIndex_r4/Constant  const=3  gui_display_data_type=Floating-point  arith_type=Floating-point  n_bits=16  bin_pt=14  preci_type=Single  exp_width=8  frac_width=24  explicit_period=off  period=Ts  equ=P=C  opselect=C  inp2=PCIN>>17  opr=+  inp1=P  carry=CIN  dbl_ovrd=off  block_type=constant
  Constant6 : xbsIndex_r4/Constant  const=1  gui_display_data_type=Floating-point  arith_type=Floating-point  n_bits=16  bin_pt=14  preci_type=Single  exp_width=8  frac_width=24  explicit_period=off  period=Ts  equ=P=C  opselect=C  inp2=PCIN>>17  opr=+  inp1=P  carry=CIN  dbl_ovrd=off  block_type=constant
  Constant7 : xbsIndex_r4/Constant  const=-3  gui_display_data_type=Floating-point  arith_type=Floating-point  n_bits=16  bin_pt=14  preci_type=Single  exp_width=8  frac_width=24  explicit_period=off  period=Ts  equ=P=C  opselect=C  inp2=PCIN>>17  opr=+  inp1=P  carry=CIN  dbl_ovrd=off  block_type=constant
  Constant8 : xbsIndex_r4/Constant  const=-1  gui_display_data_type=Floating-point  arith_type=Floating-point  n_bits=16  bin_pt=14  preci_type=Single  exp_width=8  frac_width=24  explicit_period=off  period=Ts  equ=P=C  opselect=C  inp2=PCIN>>17  opr=+  inp1=P  carry=CIN  dbl_ovrd=off  block_type=constant
  Mux : xbsIndex_r4/Mux  inputs=4  en=off  latency=1  precision=Full  arith_type=Unsigned  n_bits=16  bin_pt=14  quantization=Truncate  overflow=Wrap  dbl_ovrd=off  block_type=mux
  Mux1 : xbsIndex_r4/Mux  inputs=4  en=off  latency=1  precision=Full  arith_type=Unsigned  n_bits=16  bin_pt=14  quantization=Truncate  overflow=Wrap  dbl_ovrd=off  block_type=mux
  Out2 : Outport
  Out3 : Outport  Port=2
  wires:
  Mux1/1 -> Out3/1
  In1/1 -> BitBasher/1
  Constant1/1 -> Mux/2
  Constant2/1 -> Mux/3
  BitBasher/1 -> Mux/1
  Constant5/1 -> Mux1/2
  Constant6/1 -> Mux1/3
  Constant8/1 -> Mux1/5
  Constant7/1 -> Mux1/4
  BitBasher/2 -> Mux1/1
  Constant4/1 -> Mux/5
  Mux/1 -> Out2/1
  Constant3/1 -> Mux/4

== system Basic_DMT/Combination of Sysgen S//P and 16QAM/16-QAM 2 ==
  In1 : Inport
  BitBasher : xbsIndex_r4/BitBasher  bitexpr=|  display_expr=on  sr_1=b  arith_type1=Unsigned  bin_pt1=0  sr_2=c  arith_type2=Unsigned  bin_pt2=0  sr_3=3  arith_type3=Unsigned  bin_pt3=0  sr_4=4  arith_type4=Unsigned  bin_pt4=0  dbl_ovrd=off  block_type=bitbasher
      | b={a[3:2]}
      | c={a[1:0]}
  Constant1 : xbsIndex_r4/Constant  const=-3  gui_display_data_type=Floating-point  arith_type=Floating-point  n_bits=16  bin_pt=14  preci_type=Single  exp_width=8  frac_width=24  explicit_period=off  period=Ts  equ=P=C  opselect=C  inp2=PCIN>>17  opr=+  inp1=P  carry=CIN  dbl_ovrd=off  block_type=constant
  Constant2 : xbsIndex_r4/Constant  const=-1  gui_display_data_type=Floating-point  arith_type=Floating-point  n_bits=16  bin_pt=14  preci_type=Single  exp_width=8  frac_width=24  explicit_period=off  period=Ts  equ=P=C  opselect=C  inp2=PCIN>>17  opr=+  inp1=P  carry=CIN  dbl_ovrd=off  block_type=constant
  Constant3 : xbsIndex_r4/Constant  const=3  gui_display_data_type=Floating-point  arith_type=Floating-point  n_bits=16  bin_pt=14  preci_type=Single  exp_width=8  frac_width=24  explicit_period=off  period=Ts  equ=P=C  opselect=C  inp2=PCIN>>17  opr=+  inp1=P  carry=CIN  dbl_ovrd=off  block_type=constant
  Constant4 : xbsIndex_r4/Constant  const=1  gui_display_data_type=Floating-point  arith_type=Floating-point  n_bits=16  bin_pt=14  preci_type=Single  exp_width=8  frac_width=24  explicit_period=off  period=Ts  equ=P=C  opselect=C  inp2=PCIN>>17  opr=+  inp1=P  carry=CIN  dbl_ovrd=off  block_type=constant
  Constant5 : xbsIndex_r4/Constant  const=3  gui_display_data_type=Floating-point  arith_type=Floating-point  n_bits=16  bin_pt=14  preci_type=Single  exp_width=8  frac_width=24  explicit_period=off  period=Ts  equ=P=C  opselect=C  inp2=PCIN>>17  opr=+  inp1=P  carry=CIN  dbl_ovrd=off  block_type=constant
  Constant6 : xbsIndex_r4/Constant  const=1  gui_display_data_type=Floating-point  arith_type=Floating-point  n_bits=16  bin_pt=14  preci_type=Single  exp_width=8  frac_width=24  explicit_period=off  period=Ts  equ=P=C  opselect=C  inp2=PCIN>>17  opr=+  inp1=P  carry=CIN  dbl_ovrd=off  block_type=constant
  Constant7 : xbsIndex_r4/Constant  const=-3  gui_display_data_type=Floating-point  arith_type=Floating-point  n_bits=16  bin_pt=14  preci_type=Single  exp_width=8  frac_width=24  explicit_period=off  period=Ts  equ=P=C  opselect=C  inp2=PCIN>>17  opr=+  inp1=P  carry=CIN  dbl_ovrd=off  block_type=constant
  Constant8 : xbsIndex_r4/Constant  const=-1  gui_display_data_type=Floating-point  arith_type=Floating-point  n_bits=16  bin_pt=14  preci_type=Single  exp_width=8  frac_width=24  explicit_period=off  period=Ts  equ=P=C  opselect=C  inp2=PCIN>>17  opr=+  inp1=P  carry=CIN  dbl_ovrd=off  block_type=constant
  Mux : xbsIndex_r4/Mux  inputs=4  en=off  latency=1  precision=Full  arith_type=Unsigned  n_bits=16  bin_pt=14  quantization=Truncate  overflow=Wrap  dbl_ovrd=off  block_type=mux
  Mux1 : xbsIndex_r4/Mux  inputs=4  en=off  latency=1  precision=Full  arith_type=Unsigned  n_bits=16  bin_pt=14  quantization=Truncate  overflow=Wrap  dbl_ovrd=off  block_type=mux
  Out2 : Outport
  Out3 : Outport  Port=2
  wires:
  Mux1/1 -> Out3/1
  In1/1 -> BitBasher/1
  Constant1/1 -> Mux/2
  Constant2/1 -> Mux/3
  BitBasher/1 -> Mux/1
  Constant5/1 -> Mux1/2
  Constant6/1 -> Mux1/3
  Constant8/1 -> Mux1/5
  Constant7/1 -> Mux1/4
  BitBasher/2 -> Mux1/1
  Constant4/1 -> Mux/5
  Mux/1 -> Out2/1
  Constant3/1 -> Mux/4

== system Basic_DMT/Delay_Rem_GI/Delay_GI_DMT ==
  note: 56
  In1 : Inport
  remove_GI : Delay  DelayLength=56+56+56+56  InitialCondition=0
  Out1 : Outport
  wires:
  In1/1 -> remove_GI/1
  remove_GI/1 -> Out1/1

== system Basic_DMT/Delay_Rem_GI/Delay_GI_OFDM ==
  note: 56
  In1 : Inport
  remove_GI : Delay  DelayLength=56+56+56  InitialCondition=0
  Out1 : Outport
  wires:
  In1/1 -> remove_GI/1
  remove_GI/1 -> Out1/1

== system Basic_DMT/Delay_Rem_GI/Delay_None ==
  In1 : Inport
  Out1 : Outport
  wires:
  In1/1 -> Out1/1

== system Basic_DMT/Demodulation/Assert_Bit_Mapping ==
  In1 : Inport
  In2 : Inport  Port=2
  In3 : Inport  Port=3
  In4 : Inport  Port=4
  Add1 : Sum  Inputs=+-
  Add3 : Sum  Inputs=+-
  Check Static Range1 : simulink/Model Verification/Check  Static Range  Description=0 <= u <= 0  max=0  max_included=on  min=0  min_included=on  enabled=off  stopWhenAssertionFail=off  export=off  icon=graphic
  Check Static Range3 : simulink/Model Verification/Check  Static Range  Description=0 <= u <= 0  max=0  max_included=on  min=0  min_included=on  enabled=off  stopWhenAssertionFail=off  export=off  icon=graphic
  Delay : Delay  DelayLength=1  InitialCondition=0
  Delay1 : Delay  DelayLength=1  InitialCondition=0
  Delay4 : xbsIndex_r4/Delay  Commented=through  rst=off  infoeditControl=Selection of Reset will increase slice count due to use of real FFs and instead of SRLs  en=off  latency=3  reg_retiming=off  dbl_ovrd=off  block_type=delay
  Delay5 : xbsIndex_r4/Delay  Commented=through  rst=off  infoeditControl=Selection of Reset will increase slice count due to use of real FFs and instead of SRLs  en=off  latency=3  reg_retiming=off  dbl_ovrd=off  block_type=delay
  Gateway Out1 : xbsIndex_r4/Gateway Out  inherit_from_input=on  hdl_port=off  rows=1  columns=1  UseAsDAC=off  DACChannel='1'  interface=None  automatic_assignment=on  address_offset=hex2dec('00')  intf_description=''  timing_constraint=None  locs_specified=off  LOCs={}  io_standard={}  block_type=gatewayout
  Gateway Out2 : xbsIndex_r4/Gateway Out  inherit_from_input=on  hdl_port=off  rows=1  columns=1  UseAsDAC=off  DACChannel='1'  interface=None  automatic_assignment=on  address_offset=hex2dec('00')  intf_description=''  timing_constraint=None  locs_specified=off  LOCs={}  io_standard={}  block_type=gatewayout
  Parallel to Serial : xbsIndex_r4/Parallel to Serial  output_order=Most Significant Word First  arith_type=Unsigned  output_bits=1  bin_pt=0  rst=off  en=off  latency=1  dbl_ovrd=off  block_type=p2s
      settings: infoedit=Each sample presented at the input becomes several samples presented serially at the output.
  Parallel to Serial1 : xbsIndex_r4/Parallel to Serial  output_order=Most Significant Word First  arith_type=Unsigned  output_bits=1  bin_pt=0  rst=off  en=off  latency=1  dbl_ovrd=off  block_type=p2s
      settings: infoedit=Each sample presented at the input becomes several samples presented serially at the output.
  Scope5 : Scope  Commented=on  NumInputPorts=6
      settings: YMin=-5~-5~-5~-5~-5~-5  YMax=5~5~5~5~5~5  SaveName=ScopeData18
  Unbuffer : Unbuffer  SampleBasedProcessing=Same as frame based
  Unbuffer1 : Unbuffer  SampleBasedProcessing=Same as frame based
  wires:
  Unbuffer/1 -> Delay/1
  Delay/1 -> Scope5/1, Add3/1
  Delay1/1 -> Add1/1, Scope5/4
  Unbuffer1/1 -> Delay1/1
  Gateway Out2/1 -> Add3/2, Scope5/2
  Gateway Out1/1 -> Scope5/5, Add1/2
  Add1/1 -> Check Static Range1/1, Scope5/6
  In4/1 -> Parallel to Serial1/1
  Add3/1 -> Check Static Range3/1, Scope5/3
  In2/1 -> Unbuffer1/1
  In1/1 -> Unbuffer/1
  Parallel to Serial1/1 -> Delay5/1
  Delay5/1 -> Gateway Out1/1
  Parallel to Serial/1 -> Delay4/1
  Delay4/1 -> Gateway Out2/1
  In3/1 -> Parallel to Serial/1

== system Basic_DMT/Demodulation/Bit Demapping P1 ==
  mode : Inport
  data : Inport  Port=2
  16-QAM : Subsystem
  256-QAM : Subsystem
  Fcn : Fcn  Expr=u==0
  Fcn1 : Fcn  Expr=u==1
  Merge : Merge
  Out1 : Outport
  wires:
  data/1 -> 16-QAM/1(In1), 256-QAM/1(In1)
  Fcn/1 -> 256-QAM/Enable
  mode/1 -> Fcn1/1, Fcn/1
  Merge/1 -> Out1/1
  Fcn1/1 -> 16-QAM/Enable
  256-QAM/1(Out1) -> Merge/2
  16-QAM/1(Out1) -> Merge/1

== system Basic_DMT/Demodulation/Bit Demapping P10 ==
  mode : Inport
  data : Inport  Port=2
  16-QAM : Subsystem
  256-QAM : Subsystem
  Fcn : Fcn  Expr=u==0
  Fcn1 : Fcn  Expr=u==1
  Merge : Merge
  Out1 : Outport
  wires:
  data/1 -> 16-QAM/1(In1), 256-QAM/1(In1)
  Fcn/1 -> 256-QAM/Enable
  mode/1 -> Fcn1/1, Fcn/1
  Merge/1 -> Out1/1
  Fcn1/1 -> 16-QAM/Enable
  256-QAM/1(Out1) -> Merge/2
  16-QAM/1(Out1) -> Merge/1
